simulink model "basic_system"  (R2023b)
settings: Solver=VariableStepAuto  StartTime=0.0  StopTime=10.0  RelTol=1e-3
undefined symbols (not defined in the file or in its folder): H2, I
libraries: cstblocks x3
settings Model: Creator=lucs1  LastModifiedBy=lucs1

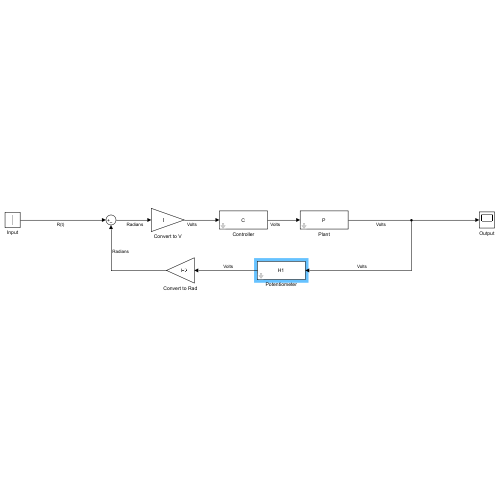
[thumbnail: Simulink's stored preview of the top-level diagram]
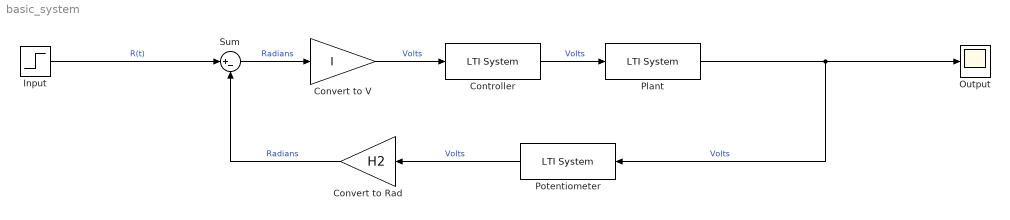
== system basic_system ==
  Controller : cstblocks/LTI System  sys=C  IC=[]  PadeOrder=0
  Convert to Rad : Gain  Gain=H2
  Convert to V : Gain  Gain=I
  Input : Step  SampleTime=0
  Output : Scope
  Plant : cstblocks/LTI System  sys=P  IC=[]  PadeOrder=0
  Potentiometer : cstblocks/LTI System  sys=H1  IC=[]  PadeOrder=0
  Sum : Sum  Inputs=|+-
  wires:
  Convert to Rad/1 -> Sum/2  "Radians"
  Sum/1 -> Convert to V/1  "Radians"
  Convert to V/1 -> Controller/1  "Volts"
  Potentiometer/1 -> Convert to Rad/1  "Volts"
  Plant/1 -> Output/1, Potentiometer/1  "Volts"
  Input/1 -> Sum/1  "R(t)"
  Controller/1 -> Plant/1  "Volts"
